simulink model "Tank_Modell_2015a"  (R2015a)
settings: Solver=ode45  StartTime=0.0  StopTime=400  MaxStep=1e-1  RelTol=1e-3
InitFcn:
  | set_parameter
values from neighbouring files (symbols this model uses):
  parInit =     [parameter_08.mat]
  parSys =     [parameter_08.mat]
undefined symbols (not defined in the file or in its folder): parSollwertfilter
libraries: simulink x3
settings Model: Creator=Wolfgang Kemmetmüller  LastModifiedBy=cds-lue-1
settings OptimizationCC: ExpressionDepthLimit=2147483647  InitFltsAndDblsToZero=on
settings DebuggingCC: SaveWithParameterizedLinksMsg=none  UnderspecifiedInitializationDetection=Classic  MergeDetectMultiDrivingBlocksExec=none  SolverPrmCheckMsg=warning  StateNameClashWarn=warning
settings SFSimCC: SimParseCustomCode=off
settings GRTTargetCC: CombineOutputUpdateFcns=off  GRTInterface=on

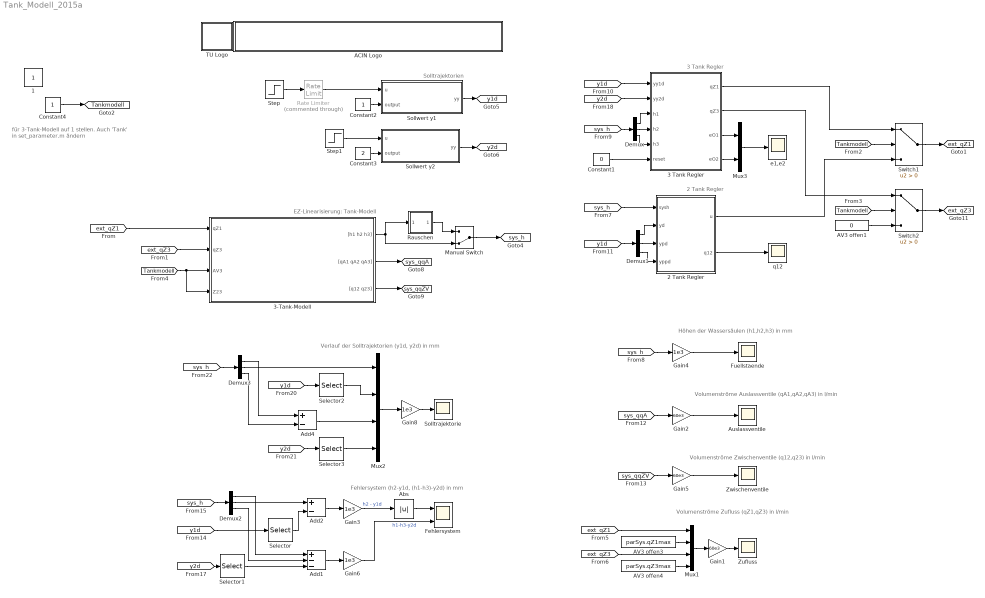
== system Tank_Modell_2015a ==
  note: Solltrajektorien
  note: 3 Tank Regler
  note: 2 Tank Regler
  note: Höhen der Wassersäulen (h1,h2,h3) in mm
  note: Volumenströme Auslassventile (qA1,qA2,qA3) in l/min
  note: Volumenströme Zwischenventile (q12,q23) in l/min
  note: Volumenströme Zufluss (qZ1,qZ3) in l/min
  note: Verlauf der Solltrajektorien (y1d, y2d) in mm
  note: Fehlersystem (h2-y1d, (h1-h3)-y2d) in mm
  note: für 3-Tank-Modell auf 1 stellen.
      | Auch 'Tank' in set_parameter.m ändern
  note: EZ-Linearisierung: Tank-Modell
  "2 Tank Regler " : MATLAB Function  TreatAsAtomicUnit=on
  3 Tank Regler : MATLAB Function  TreatAsAtomicUnit=on
  3-Tank-Modell : Subsystem
      mask init:
      | S = get_param(gcb,'UserData');
      mask Display:
      | image(S.pic);
      | port_label('input', 1, 'qZ1');
      | port_label('input', 2, 'qZ3');
      | port_label('input', 3, 'AV3');
      | port_label('input', 4, 'Z23');
      | port_label('output', 1, '[h1 h2 h3]');
      | port_label('output', 2, '[qA1 qA2 qA3]');
      | port_label('output', 3, '[q12 q23]');
  ACIN Logo : Subsystem
      mask init:
      | s = get_param(gcb,'UserData');
      mask Display:
      | image(s.logo,[0 0 439 45]);
      | %axis image
  AV3 offen1 : Constant  Value=0
  AV3 offen3 : Constant  Value=parSys.qZ1max  SampleTime=parSys.Ta
  AV3 offen4 : Constant  Value=parSys.qZ3max  SampleTime=parSys.Ta
  Abs : Abs
  Add1 : Sum  Inputs=+--
  Add2 : Sum  Inputs=+-
  Add4 : Sum  Inputs=+-
  Auslassventile : Scope
      settings: YMin=-0.19782  YMax=1.78037
  Constant1 : Constant  Value=0
  Constant2 : Constant
  Constant3 : Constant  Value=2
  Constant4 : Constant
  Demux{,1..3} (4 alike) : Demux  Outputs=3
  Fehlersystem : Scope  NumInputPorts=2
      settings: ShowLegends=on  YMin=0~0  YMax=2~6.5  SaveName=ScopeData2
  Fuellstaende : Scope
      settings: ShowLegends=on  TimeRange=400  YMin=75  YMax=275  SaveName=ScopeData3
  Gain1 : Gain  Gain=60e3
  Gain2 : Gain  Gain=60e3
  Gain{3..4,6,8} (4 alike) : Gain  Gain=1e3
  Gain5 : Gain  Gain=60e3
  Manual Switch : ManualSwitch  CurrentSetting=0
  Mux1 : Mux
  Mux2 : Mux
  Mux3 : Mux  Inputs=2
  Rate Limiter : RateLimiter  Commented=through  RisingSlewLimit=0.65/1000  FallingSlewLimit=-3/1000
  Rauschen : Subsystem
  Selector{,1..3} (4 alike) : Selector  InputPortWidth=3  Indices=[1]
  Solltrajektorie : Scope
      settings: ShowLegends=on  YMin=25  YMax=325  SaveName=ScopeData4
  Sollwert y1 : MATLAB Function  TreatAsAtomicUnit=on  SystemSampleTime=parSollwertfilter.Ta
  Sollwert y2 : MATLAB Function  TreatAsAtomicUnit=on  SystemSampleTime=parSollwertfilter.Ta
  Step : Step  Before=parSys.h2_0  After=parSys.h2_0+parSys.deltay1d  SampleTime=0
  Step1 : Step  Before=parSys.h1_0-parSys.h3_0  After=parSys.h1_0-parSys.h3_0+parSys.deltay2d  SampleTime=0
  Switch1 : Switch  Criteria=u2 > Threshold
  Switch2 : Switch  Criteria=u2 > Threshold
  TU Logo : Subsystem
      mask init:
      | s = get_param(gcb,'UserData');
      mask Display: image(s.logo,[0 0 45 45]);
  Zufluss : Scope
      settings: ShowLegends=on  YMin=0  YMax=65  SaveName=ScopeData5
  Zwischenventile : Scope
      settings: YMin=-0.20552  YMax=1.84964  SaveName=ScopeData6
  e1,e2 : Scope
      settings: ShowLegends=on  YMin=-0.0018  YMax=0.00722
  q12 : Scope
      settings: ShowLegends=on  YMin=0.000014  YMax=0.000028  SaveName=ScopeData4
  1 : Constant  IOType=siggen
  tag scope: Tankmodell=global, ext_qZ1=global, ext_qZ3=global, sys_h=global, sys_qqA=global, sys_qqZV=global, y1d=global, y2d=global
  wires:
  [sys_h] -> "2 Tank Regler "/1(sysh)
  "2 Tank Regler "/2(q12) -> q12/1
  Sollwert y1/1(yy) -> [y1d]
  Demux1/2 -> "2 Tank Regler "/3(ypd)
  Demux1/3 -> "2 Tank Regler "/4(yppd)
  [sys_h] -> Demux/1
  Demux/1 -> 3 Tank Regler/3(h1)
  Demux/2 -> 3 Tank Regler/4(h2)
  Demux/3 -> 3 Tank Regler/5(h3)
  3 Tank Regler/1(qZ1) -> Switch1/1
  3 Tank Regler/2(qZ3) -> Switch2/1
  Constant1/1 -> 3 Tank Regler/6(reset)
  [y1d] -> 3 Tank Regler/1(yy1d)
  Constant2/1 -> Sollwert y1/2(output)
  Sollwert y2/1(yy) -> [y2d]
  Constant3/1 -> Sollwert y2/2(output)
  [y2d] -> 3 Tank Regler/2(yy2d)
  Step/1 -> Rate Limiter/1
  Step1/1 -> Sollwert y2/1(u)
  3 Tank Regler/4(eO2) -> Mux3/2
  3 Tank Regler/3(eO1) -> Mux3/1
  Mux3/1 -> e1,e2/1
  Switch1/1 -> [ext_qZ1]
  Switch2/1 -> [ext_qZ3]
  "2 Tank Regler "/1(u) -> Switch1/3
  AV3 offen1/1 -> Switch2/3
  [Tankmodell] -> Switch1/2
  [Tankmodell] -> Switch2/2
  Demux1/1 -> "2 Tank Regler "/2(yd)
  [y1d] -> Demux1/1
  [sys_qqA] -> Gain2/1
  [sys_h] -> Gain4/1
  [sys_qqZV] -> Gain5/1
  [ext_qZ1] -> Mux1/1
  [ext_qZ3] -> Mux1/3
  AV3 offen4/1 -> Mux1/4
  AV3 offen3/1 -> Mux1/2
  Gain5/1 -> Zwischenventile/1
  Gain2/1 -> Auslassventile/1
  Gain4/1 -> Fuellstaende/1
  Mux1/1 -> Gain1/1
  Gain1/1 -> Zufluss/1
  [sys_h] -> Demux2/1
  Demux2/2 -> Add2/1
  Add2/1 -> Gain3/1
  Gain3/1 -> Abs/1  "h2 - y1d"
  Gain8/1 -> Solltrajektorie/1
  Demux2/1 -> Add1/1
  Demux2/3 -> Add1/2
  Add1/1 -> Gain6/1
  Gain6/1 -> Fehlersystem/2  "h1-h3-y2d"
  [y1d] -> Selector/1
  Selector/1 -> Add2/2
  [y2d] -> Selector1/1
  Selector1/1 -> Add1/3
  [sys_h] -> Demux3/1
  Demux3/1 -> Add4/1
  Demux3/3 -> Add4/2
  [y1d] -> Selector2/1
  Demux3/2 -> Mux2/1
  [y2d] -> Selector3/1
  Selector2/1 -> Mux2/2
  Add4/1 -> Mux2/3
  Selector3/1 -> Mux2/4
  Mux2/1 -> Gain8/1
  3-Tank-Modell/3("[q12 q23]") -> [sys_qqZV]
  3-Tank-Modell/2("[qA1 qA2 qA3]") -> [sys_qqA]
  Manual Switch/1 -> [sys_h]
  3-Tank-Modell/1("[h1 h2 h3]") -> Manual Switch/2, Rauschen/1(In1)
  Rauschen/1(Out1) -> Manual Switch/1
  [ext_qZ3] -> 3-Tank-Modell/2(qZ3)
  Constant4/1 -> [Tankmodell]
  [Tankmodell] -> 3-Tank-Modell/4(Z23), 3-Tank-Modell/3(AV3)
  [ext_qZ1] -> 3-Tank-Modell/1(qZ1)
  Rate Limiter/1 -> Sollwert y1/1(u)
  Abs/1 -> Fehlersystem/1

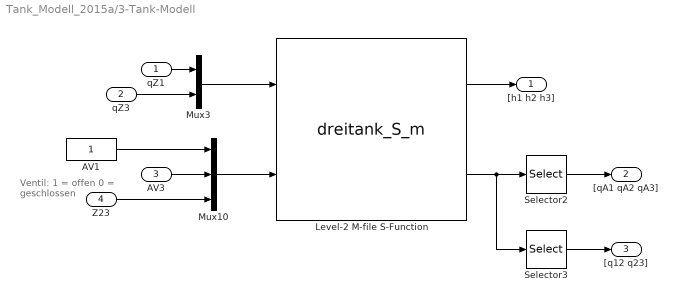
== system Tank_Modell_2015a/3-Tank-Modell ==
  note: Ventil:
      | 1 = offen
      | 0 = geschlossen
  qZ1 : Inport
  qZ3 : Inport  Port=2
  AV3 : Inport  Port=3
  Z23 : Inport  Port=4
  AV1 : Constant
  Level-2 M-file S-Function : M-S-Function  FunctionName=dreitank_S_m  Parameters=Atank, rho, eta, g, alphaA1, DA1, alphaA2, A2, alphaA3, DA3, alpha12_0, A12, Dh12, lambdac12, alpha23_0, D23, lambdac23, hmin, h1_0, h2_0, h3_0, qZ1max, qZ3max, flaglimqZ, h_max, h_min  mask{Atank=parSys.Atank, rho=parSys.rho, eta=parSys.eta, g=parSys.g, alphaA1=parSys.alphaA1, DA1=parSys.DA1*parSys.DA1_Abw, alphaA2=parSys.alphaA2, A2=parSys.A2, alphaA3=parSys.alphaA3, DA3=parSys.DA3*parSys.DA3_Abw, alpha12_0=parSys.alpha12_0, A12=parSys.A12, Dh12=parSys.Dh12, lambdac12=parSys.lambdac12, alpha23_0=parSys.alpha23_0, D23=parSys.D23, lambdac23=parSys.lambdac23, hmin=parSys.hmin, h1_0=parSys.h1_0, h2_0=parSys.h2_0, h3_0=parSys.h3_0, qZ1max=parSys.qZ1max, qZ3max=parSys.qZ3max, h_max=parSys.hmax, h_min=parSys.hmin, flaglimqZ=on}
      mask prompts: Atank "Grundfläche Tank (Atank)"; rho "Dichte Wasser (rho)"; eta "Viskosität Wasser (eta)"; g "Gravitationskonstante (g)"; alphaA1 "Kontraktionskoeffizient AV1 (alphaA1)"; DA1 "Durchmesser AV1 (DA1)"; alphaA2 "Kontraktionskoeffizient AV2 (alphaA2)"; A2 "Querschnittsfläche AV2 (A2)"; alphaA3 "Kontraktionskoeffizient AV3 (alphaA3)"; DA3 "Durchmesser A3 (DA3)"; alpha12_0 "Kontraktionskoeffizient ZV12 (alpha12_0)"; A12 "Querschnittsfläche ZV12 (A12)"; Dh12 "hydraulischer Durchmesser ZV12 (Dh12)"; lambdac12 "kritische Fließzahl ZV12 (lambdac12)"; alpha23_0 "Kontraktionskoeffizient ZV23 (alpha23_0)"; D23 "Durchmesser ZV23 (D23)"; lambdac23 "kritische Fließzahl ZV23 (lambdac23)"; hmin "minimale Füllhöhe (hmin)"; h1_0 "Anfangsbedingung h1 (h1_0)"; h2_0 "Anfangsbedingung h2 (h2_0)"; h3_0 "Anfangsbedingung h3 (h3_0)"; qZ1max "maximaler Zufluss Z1 (qZ1max)"; qZ3max "maximaler Zufluss Z3 (qZ3max)"; h_max "Maximale Füllhöhe"; h_min "Minimale Füllhöhe"; flaglimqZ "Beschränkung der Zuflüsse ein"
      mask Display:
      | port_label('input',1,'Zulaufvolumenströme')
      | port_label('input',2,'Zustand Ventile')
      | 
      | port_label('output',1,'Zustände')
      | port_label('output',2,'Volumenströme')
  Mux10 : Mux  Inputs=3
  Mux3 : Mux  Inputs=2
  Selector2 : Selector  InputPortWidth=5  Indices=[1 2 3]
  Selector3 : Selector  InputPortWidth=5  Indices=[4 5]
  "[h1 h2 h3]" : Outport
  "[qA1 qA2 qA3]" : Outport  Port=2
  "[q12 q23]" : Outport  Port=3
  wires:
  AV1/1 -> Mux10/1
  Mux3/1 -> Level-2 M-file S-Function/1
  Mux10/1 -> Level-2 M-file S-Function/2
  qZ1/1 -> Mux3/1
  Level-2 M-file S-Function/1 -> "[h1 h2 h3]"/1
  qZ3/1 -> Mux3/2
  Level-2 M-file S-Function/2 -> Selector2/1, Selector3/1
  Selector2/1 -> "[qA1 qA2 qA3]"/1
  Selector3/1 -> "[q12 q23]"/1
  Z23/1 -> Mux10/3
  AV3/1 -> Mux10/2

== system Tank_Modell_2015a/ACIN Logo ==

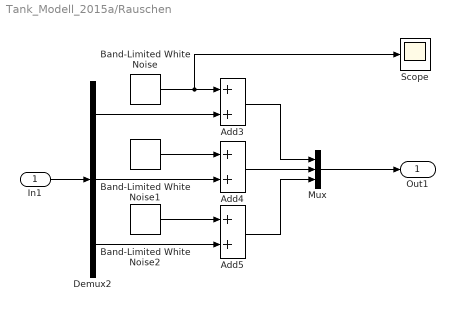
== system Tank_Modell_2015a/Rauschen ==
  In1 : Inport
  Add3 : Sum
  Add4 : Sum
  Add5 : Sum
  Band-Limited White Noise : simulink/Sources/Band-Limited White Noise  Cov=[2.5e-10]  Ts=parSys.Ta  seed=[23341]
  Band-Limited White Noise1 : simulink/Sources/Band-Limited White Noise  Cov=[2.5e-10]  Ts=parSys.Ta  seed=[32464]
  Band-Limited White Noise2 : simulink/Sources/Band-Limited White Noise  Cov=[2.5e-10]  Ts=parSys.Ta  seed=[98543]
  Demux2 : Demux  Outputs=3
  Mux : Mux  Inputs=3
  Scope : Scope
      settings: YMin=-0.00016  YMax=0.00017
  Out1 : Outport
  wires:
  Add5/1 -> Mux/3
  Band-Limited White Noise/1 -> Scope/1, Add3/1
  Demux2/1 -> Add3/2
  Add4/1 -> Mux/2
  Add3/1 -> Mux/1
  Demux2/2 -> Add4/2
  Mux/1 -> Out1/1
  Band-Limited White Noise1/1 -> Add4/1
  In1/1 -> Demux2/1
  Band-Limited White Noise2/1 -> Add5/1
  Demux2/3 -> Add5/2

== system Tank_Modell_2015a/TU Logo ==

== matlab function Tank_Modell_2015a/Sollwert y1 ==
  settings: updateMethod=DISCRETE  sampleTime=parSollwertfilter.Ta
  data: u input; output input; yy output; parSollwertfilter parameter; parSys parameter
function yy  = sollwertfilter(u, output, parSollwertfilter, parSys)
persistent x;
% Anfangswert abziehen
if output < 1.5
    % 2-Tank
    u = u-parSys.h2_0; 
else
    % 3-Tank
    u = u-parSys.h1_0+parSys.h3_0;
end

a=parSollwertfilter.a;
b=parSollwertfilter.b;
c=parSollwertfilter.c;
d=parSollwertfilter.d;

if(isempty(x))
    x0_Filter=parSollwertfilter.x0_Filter;
    x=x0_Filter;
end

yt=c*x+d*u;

% Anfangswert wieder addieren
if output < 1.5
    % 2-Tank
    y=yt(1)+parSys.h2_0; 
else
    % 3-Tank
    y=yt(1)+parSys.h1_0-parSys.h3_0; 
end
yp=yt(2);
ypp=yt(3);

yy = [y; yp; ypp];

x=a*x+b*u;

== matlab function Tank_Modell_2015a/2 Tank Regler  ==
  settings: updateMethod=DISCRETE  sampleTime=parSys.Ta
  data: u output; sysh input; parSys parameter; yd input; ypd input; yppd input; q12 output; parInit parameter
function [u,q12]  = fcn(sysh, parSys, yd, ypd, yppd, parInit)

Atank = parSys.Atank;
rho = parSys.rho;
eta = parSys.eta;
g = parSys.g;
alphaA1 = parSys.alphaA1;
DA1 = parSys.DA1;
alphaA2 = parSys.alphaA2;
A2 = parSys.A2;
alphaA3 = parSys.alphaA3;
DA3 = parSys.DA3;
alpha12_0 = parSys.alpha12_0;
A12 = parSys.A12;
Dh12 = parSys.Dh12;
lambdac12 = parSys.lambdac12;
alpha23_0 = parSys.alpha23_0;
D23 = parSys.D23;
lambdac23 = parSys.lambdac23;
hmin = parSys.hmin;
hmax = parSys.hmax;
dh12min = parSys.dh12min;
a0 = parInit.a0;
a1 = parInit.a1;

h1=sysh(1);
h2=sysh(2);
qA1 = alphaA1 * DA1 ^ 2 * pi * sqrt(0.2e1) * sqrt(g) * sqrt(h1) / 0.4e1;
qA2 = alphaA2 * A2 * sqrt(0.2e1) * sqrt(g) * sqrt(h2);

dqA2_dh2 = alphaA2 * A2 * sqrt(0.2e1) * sqrt(g) * h2 ^ (-0.1e1 / 0.2e1) / 0.2e1;

if abs(h1-h2) > dh12min
    dq12_dh1 = 0.2e1 * alpha12_0 * Dh12 * rho / eta * g / lambdac12 * (0.1e1 - tanh(0.2e1 * Dh12 * rho / eta * sqrt(0.2e1) * sqrt(g) * sqrt(abs(h1 - h2)) / lambdac12) ^ 2) * A12 + alpha12_0 * tanh(0.2e1 * Dh12 * rho / eta * sqrt(0.2e1) * sqrt(g) * sqrt(abs(h1 - h2)) / lambdac12) * A12 * sqrt(0.2e1) * sqrt(g) * (abs(h1 - h2) ^ (-0.1e1 / 0.2e1)) / 0.2e1;
    dq12_dh2 = -0.2e1 * alpha12_0 * Dh12 * rho / eta * g / lambdac12 * (0.1e1 - tanh(0.2e1 * Dh12 * rho / eta * sqrt(0.2e1) * sqrt(g) * sqrt(abs(h1 - h2)) / lambdac12) ^ 2) * A12 - alpha12_0 * tanh(0.2e1 * Dh12 * rho / eta * sqrt(0.2e1) * sqrt(g) * sqrt(abs(h1 - h2)) / lambdac12) * A12 * sqrt(0.2e1) * sqrt(g) * (abs(h1 - h2) ^ (-0.1e1 / 0.2e1)) / 0.2e1;
else
    %Linearisierung
    dq12_dh1 = parSys.d_dq12_dh1 + parSys.k_dq12_dh1*abs(h1-h2);
    dq12_dh2 = parSys.d_dq12_dh2 + parSys.k_dq12_dh2*abs(h1-h2);
end
q12 = alpha12_0 * tanh(0.2e1 * Dh12 * rho / eta * sqrt(0.2e1) * sqrt(g) * sqrt(abs(h1 - h2)) / lambdac12) * A12 * sqrt(0.2e1) * sqrt(g) * sqrt(abs(h1 - h2)) * sign((h1 - h2));

u = 0.1e1 / dq12_dh1 * Atank ^ 2 * (yppd - dq12_dh1 / Atank ^ 2 * (-q12 - qA1) - (dq12_dh2 - dqA2_dh2) / Atank ^ 2 * (q12 - qA2) - a0 * (h2 - yd) - a1 * ((q12 - qA2) / Atank - ypd));

== matlab function Tank_Modell_2015a/3 Tank Regler ==
  settings: updateMethod=DISCRETE  sampleTime=parSys.Ta
  data: qZ1 output; qZ3 output; yy1d input; yy2d input; h1 input; h2 input; h3 input; reset input; parSys parameter; parInit parameter; eO1 output; eO2 output
function [qZ1,qZ3,eO1,eO2]  = fcn(yy1d, yy2d, h1, h2, h3, reset, parSys, parInit)

persistent e1
persistent e2

if isempty(e1)
    e1 = 0;
end

if isempty(e2)
    e2 = 0;
end

if reset
    e1 = 0;
    e2 = 0;
end
    

Atank = parSys.Atank;
rho = parSys.rho;
eta = parSys.eta;
g = parSys.g;
alphaA1 = parSys.alphaA1;
DA1 = parSys.DA1;
alphaA2 = parSys.alphaA2;
A2 = parSys.A2;
alphaA3 = parSys.alphaA3;
DA3 = parSys.DA3;
alpha12_0 = parSys.alpha12_0;
A12 = parSys.A12;
Dh12 = parSys.Dh12;
lambdac12 = parSys.lambdac12;
alpha23_0 = parSys.alpha23_0;
D23 = parSys.D23;
lambdac23 = parSys.lambdac23;
hmin = parSys.hmin;
hmax = parSys.hmax;
dh12min = parSys.dh12min;
a0 = parInit.a0;
a1 = parInit.a1;
dh23min = parSys.dh12min;

A3 = DA3^2*pi/4;
%laut angabe
Dh23 = D23;
A23 = D23^2*pi/4;

y1dpp = yy1d(3);
y1dp  = yy1d(2);
y1d   = yy1d(1);

y2dp  = yy2d(2);
y2d   = yy2d(1);


qA1 = alphaA1 * DA1 ^ 2 * pi * sqrt(0.2e1) * sqrt(g) * sqrt(h1) / 0.4e1;
qA2 = alphaA2 * A2 * sqrt(0.2e1) * sqrt(g) * sqrt(h2);
qA3 = alphaA3 * DA3 ^ 2 * pi * sqrt(0.2e1) * sqrt(g) * sqrt(h3) / 0.4e1;


dqA2_dh2 = alphaA2 * A2 * sqrt(0.2e1) * sqrt(g) * h2 ^ (-0.1e1 / 0.2e1) / 0.2e1;

if abs(h1-h2) > dh12min
    dq12_dh1 = 0.2e1 * alpha12_0 * Dh12 * rho / eta * g / lambdac12 * (0.1e1 - tanh(0.2e1 * Dh12 * rho / eta * sqrt(0.2e1) * sqrt(g) * sqrt(abs(h1 - h2)) / lambdac12) ^ 2) * A12 + alpha12_0 * tanh(0.2e1 * Dh12 * rho / eta * sqrt(0.2e1) * sqrt(g) * sqrt(abs(h1 - h2)) / lambdac12) * A12 * sqrt(0.2e1) * sqrt(g) * (abs(h1 - h2) ^ (-0.1e1 / 0.2e1)) / 0.2e1;
    dq12_dh2 = -0.2e1 * alpha12_0 * Dh12 * rho / eta * g / lambdac12 * (0.1e1 - tanh(0.2e1 * Dh12 * rho / eta * sqrt(0.2e1) * sqrt(g) * sqrt(abs(h1 - h2)) / lambdac12) ^ 2) * A12 - alpha12_0 * tanh(0.2e1 * Dh12 * rho / eta * sqrt(0.2e1) * sqrt(g) * sqrt(abs(h1 - h2)) / lambdac12) * A12 * sqrt(0.2e1) * sqrt(g) * (abs(h1 - h2) ^ (-0.1e1 / 0.2e1)) / 0.2e1;
else
    %Linearisierung
    dq12_dh1 = parSys.d_dq12_dh1 + parSys.k_dq12_dh1*abs(h1-h2);
    dq12_dh2 = parSys.d_dq12_dh2 + parSys.k_dq12_dh2*abs(h1-h2);
end

if abs(h2-h3) > dh23min
    dq23_dh2 = alpha23_0 * D23 ^ 3 * rho / eta * g / lambdac23 * (0.1e1 - tanh(0.2e1 * D23 * rho / eta * sqrt(0.2e1) * sqrt(g) * sqrt(abs(h2 - h3)) / lambdac23) ^ 2) * pi / 0.2e1 + alpha23_0 * tanh(0.2e1 * D23 * rho / eta * sqrt(0.2e1) * sqrt(g) * sqrt(abs(h2 - h3)) / lambdac23) * D23 ^ 2 * pi * sqrt(0.2e1) * sqrt(g) * (abs(h2 - h3) ^ (-0.1e1 / 0.2e1)) / 0.8e1;
    dq23_dh3 = -alpha23_0 * D23 ^ 3 * rho / eta * g / lambdac23 * (0.1e1 - tanh(0.2e1 * D23 * rho / eta * sqrt(0.2e1) * sqrt(g) * sqrt(abs(h2 - h3)) / lambdac23) ^ 2) * pi / 0.2e1 - alpha23_0 * tanh(0.2e1 * D23 * rho / eta * sqrt(0.2e1) * sqrt(g) * sqrt(abs(h2 - h3)) / lambdac23) * D23 ^ 2 * pi * sqrt(0.2e1) * sqrt(g) * (abs(h2 - h3) ^ (-0.1e1 / 0.2e1)) / 0.8e1;
else
    %Linearisierung
    dq23_dh2 = parSys.d_dq23_dh2 + parSys.k_dq23_dh2*abs(h2-h3);
    dq23_dh3 = parSys.d_dq23_dh3 + parSys.k_dq23_dh3*abs(h2-h3);
end

q12 = alpha12_0 * tanh(0.2e1 * Dh12 * rho / eta * sqrt(0.2e1) * sqrt(g) * sqrt(abs(h1 - h2)) / lambdac12) * A12 * sqrt(0.2e1) * sqrt(g) * sqrt(abs(h1 - h2)) * sign((h1 - h2));
q23 = alpha23_0 * tanh(0.2e1 * D23 * rho / eta * sqrt(0.2e1) * sqrt(g) * sqrt(abs(h2 - h3)) / lambdac23) * D23 ^ 2 * pi * sqrt(0.2e1) * sqrt(g) * sqrt(abs(h2 - h3)) * sign((h2 - h3)) / 0.4e1;

Lf1h1 = (q12 - q23 - qA2) / Atank;
Lf2h1 = dq12_dh1 / Atank ^ 2 * (-q12 - qA1) + (dq12_dh2 - dq23_dh2 - dqA2_dh2) / Atank ^ 2 * (q12 - q23 - qA2) - dq23_dh3 / Atank ^ 2 * (q23 - qA3);
Lg1Lf1h1 = dq12_dh1 / Atank ^ 2;
Lg2Lf1h1 = -dq23_dh3 / Atank ^ 2;
Lg1h2 = 0.1e1 / Atank;
Lg2h2 = -0.1e1 / Atank;
Lf1h2 = (-q12 - qA1) / Atank - (q23 - qA3) / Atank;

% v um I-Anteil schon erweitert
v = [y1dpp - parInit.a10 * (h2 - y1d) - parInit.a11 * (Lf1h1 - y1dp) - parInit.a1I * e1;
     y2dp  - parInit.a20 * (h1 - h3 - y2d) - parInit.a2I * e2
     ];

bb = [Lf2h1; Lf1h2;];
DD_inv = [-Lg2h2 / (Lg1h2 * Lg2Lf1h1 - Lg2h2 * Lg1Lf1h1) Lg2Lf1h1 / (Lg1h2 * Lg2Lf1h1 - Lg2h2 * Lg1Lf1h1); Lg1h2 / (Lg1h2 * Lg2Lf1h1 - Lg2h2 * Lg1Lf1h1) -Lg1Lf1h1 / (Lg1h2 * Lg2Lf1h1 - Lg2h2 * Lg1Lf1h1);];
u_temp = DD_inv*(-bb+v);
qZ1 = u_temp(1);
qZ3 = u_temp(2);

%Anti-Windup
if qZ1 < parSys.qZ1max && qZ1 > parSys.qZ1min && qZ3 < parSys.qZ3max && qZ3 > parSys.qZ3min
    e1 = e1 + (h2 - y1d)*parSys.Ta;
    e2 = e2 + (h1 - h3 - y2d)*parSys.Ta;
end

eO1 = e1;
eO2 = e2;

end

== matlab function Tank_Modell_2015a/Sollwert y2 ==
  settings: updateMethod=DISCRETE  sampleTime=parSollwertfilter.Ta
  data: u input; output input; yy output; parSollwertfilter parameter; parSys parameter
function yy  = sollwertfilter(u, output, parSollwertfilter, parSys)
persistent x;
% Anfangswert abziehen
if output < 1.5
    % 2-Tank
    u = u-parSys.h2_0; 
else
    % 3-Tank
    u = u-parSys.h1_0+parSys.h3_0;
end

a=parSollwertfilter.a;
b=parSollwertfilter.b;
c=parSollwertfilter.c;
d=parSollwertfilter.d;

if(isempty(x))
    x0_Filter=parSollwertfilter.x0_Filter;
    x=x0_Filter;
end

yt=c*x+d*u;

% Anfangswert wieder addieren
if output < 1.5
    % 2-Tank
    y=yt(1)+parSys.h2_0; 
else
    % 3-Tank
    y=yt(1)+parSys.h1_0-parSys.h3_0; 
end
yp=yt(2);
ypp=yt(3);

yy = [y; yp; ypp];

x=a*x+b*u;
